simulink model "SimplePID"  (R2025b)
settings: Solver=ode4  StartTime=0.0  StopTime=10.0  FixedStep=0.001  RelTol=1e-3
settings Model: Creator=sputnik  LastModifiedBy=sputnik

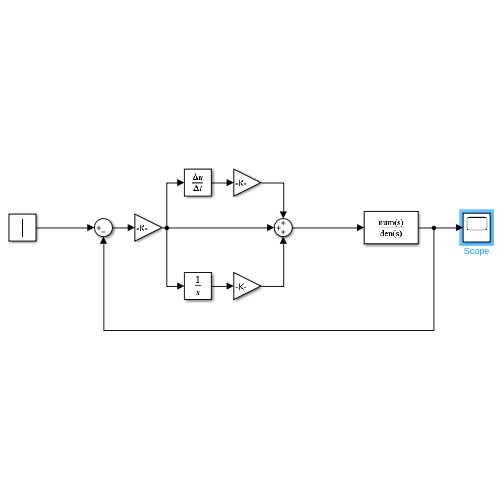
[thumbnail: Simulink's stored preview of the top-level diagram]
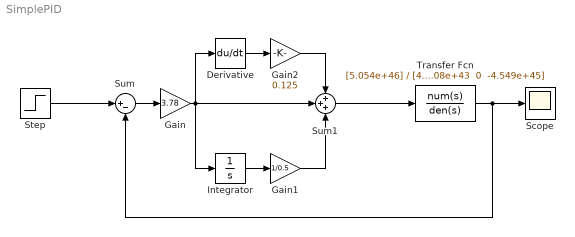
== system SimplePID ==
  Derivative : Derivative
  Gain : Gain  Gain=3.78
  Gain1 : Gain  Gain=1/0.5
  Gain2 : Gain  Gain=0.125
  Integrator : Integrator
  Scope : Scope
      settings: ActiveDisplayYMinimum=-0.27395030957425381  ActiveDisplayYMaximum=1.312813853904929
  Step : Step  Time=5  Before=1  After=0  SampleTime=0
  Sum : Sum  Inputs=|+-
  Sum1 : Sum  Inputs=+++
  Transfer Fcn : TransferFcn  Numerator=[5.054e+46]  Denominator="[4.308e+43  0  -4.549e+45]"
  wires:
  Step/1 -> Sum/1
  Transfer Fcn/1 -> Sum/2, Scope/1
  Sum1/1 -> Transfer Fcn/1
  Sum/1 -> Gain/1
  Integrator/1 -> Gain1/1
  Gain/1 -> Derivative/1, Integrator/1, Sum1/2
  Gain1/1 -> Sum1/3
  Derivative/1 -> Gain2/1
  Gain2/1 -> Sum1/1
